simulink model "Gray_Binarization"  (R2013b)
settings: Solver=ode45  StartTime=0.0  StopTime=1000  RelTol=1e-3
InitFcn:
  | %% DSPBuilder Start
  | alt_dspbuilder_update_model(bdroot)
  | %% DSPBuilder End
libraries: allblocks_alteradspbuilder2 x44, simulink x3
settings Model: Creator=Given_Jiang  LastModifiedBy=Given_Jiang

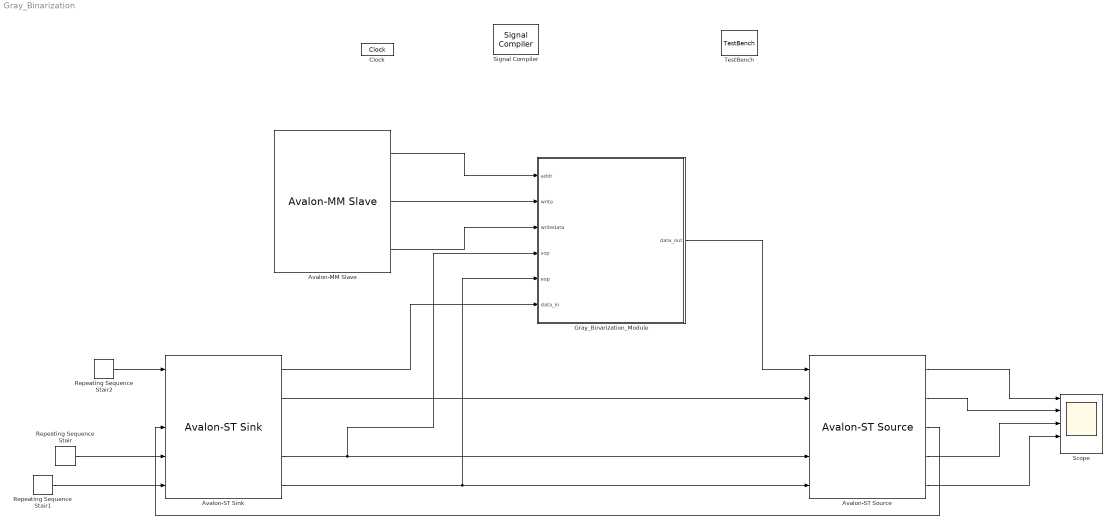
== system Gray_Binarization ==
  Avalon-MM Slave : allblocks_alteradspbuilder2/Avalon-MM Slave  iofile=E:\FPGA\SOC\Quartus\quartus\dsp_builder\design\VIP_LIB\Gray_Binarization\tb_Gray_Binarization\Gray%5FBinarization_Avalon-MM+Slave_address.salt,E:\FPGA\SOC\Quartus\quartus\dsp_builder\design\VIP_LIB\Gray_Binarization\tb_Gray_Binarization\Gray%5FBinarization_Avalon-MM+Slave_write.salt,E:\FPGA\SOC\Quartus\quartus\dsp_builder\design\VIP_LIB\Gray_Binarization\tb_Gray_Binarization\Gray%5FBinarization_Avalon-MM+Slave_writedata.salt,  SpecifyClock=off  addrWidth=2  addrAlignment=Dynamic  addrType=Write  BusType=Unsigned Integer  bwl=32  bwr=0  byteEnable=off  flowCtrl=off  pipeline=off  waitStateFormat=Fixed  readWaitStateCycles=0  writeWaitStateCycles=1  readLatencyFormat=Fixed  readLatencyCycles=0  burst=off  maxBurst=4  irq=off  receiveBeginTransfer=off  useChipSelect=off  externalType=Inferred  PORTTYPE=Output
  Avalon-ST Sink : allblocks_alteradspbuilder2/Avalon-ST Sink  iofile=E:\FPGA\SOC\Quartus\quartus\dsp_builder\design\VIP_LIB\Gray_Binarization\tb_Gray_Binarization\Gray%5FBinarization_Avalon-ST+Sink_data.salt,E:\FPGA\SOC\Quartus\quartus\dsp_builder\design\VIP_LIB\Gray_Binarization\tb_Gray_Binarization\Gray%5FBinarization_Avalon-ST+Sink_valid.salt,E:\FPGA\SOC\Quartus\quartus\dsp_builder\design\VIP_LIB\Gray_Binarization\tb_Gray_Binarization\Gray%5FBinarization_Avalon-ST+Sink_ready.capture,E:\FPGA\SOC\Quartus\quartus\dsp_builder\design\VIP_LIB\Gray_Binarization\tb_Gray_Binarization\Gray%5FBinarization_Avalon-ST+Sink_startofpacket.salt,E:\FPGA\SOC\Quartus\quartus\dsp_builder\design\VIP_LIB\Gray_Binarization\tb_Gray_Binarization\Gray%5FBinarization_Avalon-ST+Sink_endofpacket.salt,  SpecifyClock=off  BusType=Unsigned Integer  bwl=24  bwr=0  symbolWidth=8  symbolsPerBeat=3  numOfChannels=0  numOfErrorDescriptors=0  endOfPacket=on  startOfPacket=on  empty=off  readyLatency=1  externalType=Inferred  PORTTYPE=Output
  Avalon-ST Source : allblocks_alteradspbuilder2/Avalon-ST Source  iofile=E:\FPGA\SOC\Quartus\quartus\dsp_builder\design\VIP_LIB\Gray_Binarization\tb_Gray_Binarization\Gray%5FBinarization_Avalon-ST+Source_data.capture,E:\FPGA\SOC\Quartus\quartus\dsp_builder\design\VIP_LIB\Gray_Binarization\tb_Gray_Binarization\Gray%5FBinarization_Avalon-ST+Source_valid.capture,E:\FPGA\SOC\Quartus\quartus\dsp_builder\design\VIP_LIB\Gray_Binarization\tb_Gray_Binarization\Gray%5FBinarization_Avalon-ST+Source_ready.salt,E:\FPGA\SOC\Quartus\quartus\dsp_builder\design\VIP_LIB\Gray_Binarization\tb_Gray_Binarization\Gray%5FBinarization_Avalon-ST+Source_startofpacket.capture,E:\FPGA\SOC\Quartus\quartus\dsp_builder\design\VIP_LIB\Gray_Binarization\tb_Gray_Binarization\Gray%5FBinarization_Avalon-ST+Source_endofpacket.capture,  SpecifyClock=off  BusType=Unsigned Integer  bwl=24  bwr=0  symbolWidth=8  symbolsPerBeat=3  numOfChannels=0  numOfErrorDescriptors=0  endOfPacket=on  startOfPacket=on  empty=off  readyLatency=1  externalType=Inferred  PORTTYPE=Input
  Clock : allblocks_alteradspbuilder2/Clock  ClockPeriod=7.5  ClockPeriodUnit=ns  SampleTime=1  ResetLatency=0  ResetRegisterCascadeDepth=0  SimulationStartCycle=5  PhaseOffset=0  Reset=aclr  ResetType=Active Low  Export=off
  Gray_Binarization_Module : Subsystem
  Repeating Sequence Stair : simulink/Sources/Repeating Sequence Stair  OutValues=[1 0 0 0 1 0 0 0 0 0].'  tsamp=-1  OutMin=[]  OutMax=[]  OutDataTypeStr=double  OutputDataTypeScalingMode=double  OutDataType=fixdt(0,8)  ConRadixGroup=Best Precision: Vector-wise  OutScaling=2^-12
  Repeating Sequence Stair1 : simulink/Sources/Repeating Sequence Stair  OutValues=[0 0 0 1 0 0 0 0 0 1].'  tsamp=-1  OutMin=[]  OutMax=[]  OutDataTypeStr=double  OutputDataTypeScalingMode=double  OutDataType=fixdt(0,8)  ConRadixGroup=Best Precision: Vector-wise  OutScaling=2^-12
  Repeating Sequence Stair2 : simulink/Sources/Repeating Sequence Stair  OutValues=[15 101 102 103 0 65793 66305 255 255 1].'  tsamp=-1  OutMin=[]  OutMax=[]  OutDataTypeStr=double  OutputDataTypeScalingMode=double  OutDataType=fixdt(0,8)  ConRadixGroup=Best Precision: Vector-wise  OutScaling=2^-12
  Scope : Scope  NumInputPorts=5
      settings: YMin=-5~-5~-5~-5~-5  YMax=5~5~5~5~5
  Signal Compiler : allblocks_alteradspbuilder2/Signal Compiler  DeviceFamily=Cyclone V  DeviceName=AUTO  DisableEarlyHDLGeneration=off  EnableSignalTap=off  SignalTapDepth=128  UseBoardBlock=off  StpUseDefaultClock=on  StpClock=Clock  ExportDir=E:\FPGA\SOC\Quartus\quartus\dsp_builder
  TestBench : allblocks_alteradspbuilder2/TestBench  enable=on  advancedMode=on  modelSimGui=on  maxDisplayErrors=10  mismatchErrorLevel=Error  simdatafile=E:\FPGA\SOC\Quartus\quartus\dsp_builder\design\VIP_LIB\Gray_Binarization\tb_Gray_Binarization\Gray_Binarization.simdata.tcl
  wires:
  Avalon-ST Sink/2 -> Avalon-ST Source/2
  Avalon-ST Source/3 -> Avalon-ST Sink/3
  Avalon-ST Sink/4 -> Gray_Binarization_Module/4(sop), Avalon-ST Source/4
  Avalon-ST Sink/5 -> Gray_Binarization_Module/5(eop), Avalon-ST Source/5
  Avalon-ST Sink/1 -> Gray_Binarization_Module/6(data_in)
  Avalon-MM Slave/1 -> Gray_Binarization_Module/1(addr)
  Avalon-MM Slave/2 -> Gray_Binarization_Module/2(write)
  Avalon-MM Slave/3 -> Gray_Binarization_Module/3(writedata)
  Gray_Binarization_Module/1(data_out) -> Avalon-ST Source/1
  Repeating Sequence Stair/1 -> Avalon-ST Sink/4
  Repeating Sequence Stair1/1 -> Avalon-ST Sink/5
  Repeating Sequence Stair2/1 -> Avalon-ST Sink/1
  Avalon-ST Source/1 -> Scope/1
  Avalon-ST Source/2 -> Scope/2
  Avalon-ST Source/4 -> Scope/3
  Avalon-ST Source/5 -> Scope/4

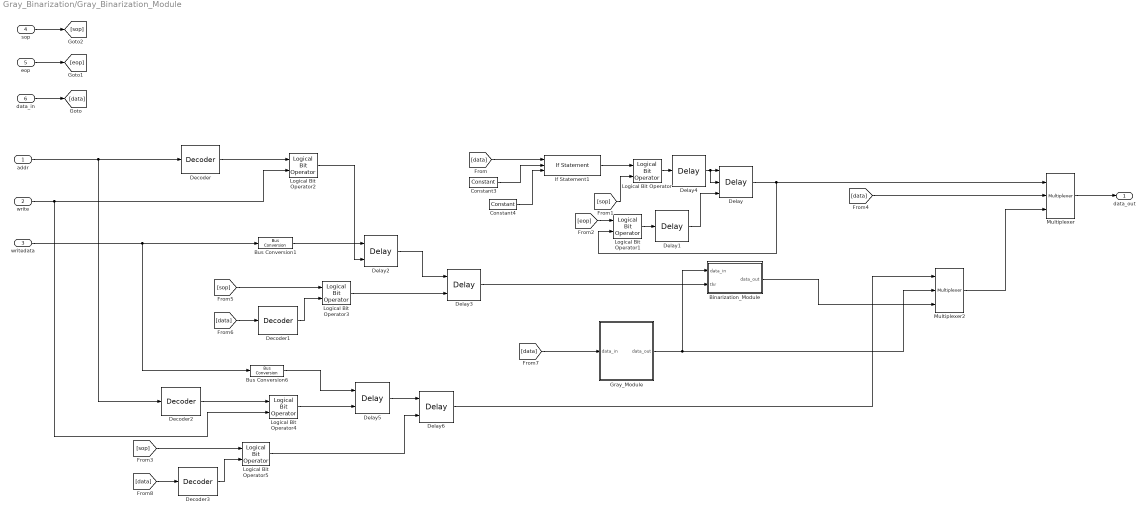
== system Gray_Binarization/Gray_Binarization_Module ==
  addr : Inport
  write : Inport  Port=2
  writedata : Inport  Port=3
  sop : Inport  Port=4
  eop : Inport  Port=5
  data_in : Inport  Port=6
  Binarization_Module : Subsystem
  Bus Conversion1 : allblocks_alteradspbuilder2/Bus Conversion  BusType=Unsigned Integer  ibwl=32  ibwr=1  bwl=8  bwr=1  bitToConnectToOutputLSB=0  round=off  saturate=off  pipeline_display=0
  Bus Conversion6 : allblocks_alteradspbuilder2/Bus Conversion  BusType=Unsigned Integer  ibwl=32  ibwr=1  bwl=1  bwr=1  bitToConnectToOutputLSB=0  round=off  saturate=off  pipeline_display=0
  Constant3 : allblocks_alteradspbuilder2/Constant  mask_cst=0  BusType=Unsigned Integer  bwl=24  bwr=0  roundMode=Truncate  satMode=Wrap  SpecifyClock=off  allowFloatingPointOverride=on  logOutputs=off  logFile=E:\FPGA\SOC\Quartus\quartus\dsp_builder\design\VIP_LIB\Gray_Binarization\tb_Gray_Binarization\Gray%5FBinarization_Gray%5FBinarization%5FModule_Constant3.fixedpointlog
  Constant4 : allblocks_alteradspbuilder2/Constant  mask_cst=15  BusType=Unsigned Integer  bwl=24  bwr=0  roundMode=Truncate  satMode=Wrap  SpecifyClock=off  allowFloatingPointOverride=on  logOutputs=off  logFile=E:\FPGA\SOC\Quartus\quartus\dsp_builder\design\VIP_LIB\Gray_Binarization\tb_Gray_Binarization\Gray%5FBinarization_Gray%5FBinarization%5FModule_Constant4.fixedpointlog
  Decoder : allblocks_alteradspbuilder2/Decoder  BusType=Unsigned Integer  bwl=2  bwr=2  registered=on  pipeline_display=1  value=2
  Decoder1 : allblocks_alteradspbuilder2/Decoder  BusType=Unsigned Integer  bwl=24  bwr=2  registered=off  pipeline_display=0  value=15
  Decoder2 : allblocks_alteradspbuilder2/Decoder  BusType=Unsigned Integer  bwl=2  bwr=2  registered=on  pipeline_display=1  value=1
  Decoder3 : allblocks_alteradspbuilder2/Decoder  BusType=Unsigned Integer  bwl=24  bwr=2  registered=off  pipeline_display=0  value=15
  Delay : allblocks_alteradspbuilder2/Delay  pipeline=1  pipeline_display=1  ClockPhase=1  use_ena=on  use_sclr=on  allowFloatingPointOverride=on  logOutputs=off  logFile=E:\FPGA\SOC\Quartus\quartus\dsp_builder\design\VIP_LIB\Gray_Binarization\tb_Gray_Binarization\Gray%5FBinarization_Gray%5FBinarization%5FModule_Delay.fixedpointlog  use_init=on  reset_value=0
  Delay1 : allblocks_alteradspbuilder2/Delay  pipeline=1  pipeline_display=1  ClockPhase=1  use_ena=off  use_sclr=off  allowFloatingPointOverride=on  logOutputs=off  logFile=E:\FPGA\SOC\Quartus\quartus\dsp_builder\design\VIP_LIB\Gray_Binarization\tb_Gray_Binarization\Gray%5FBinarization_Gray%5FBinarization%5FModule_Delay1.fixedpointlog  use_init=off  reset_value=0
  Delay2 : allblocks_alteradspbuilder2/Delay  pipeline=1  pipeline_display=1  ClockPhase=1  use_ena=on  use_sclr=off  allowFloatingPointOverride=on  logOutputs=off  logFile=E:\FPGA\SOC\Quartus\quartus\dsp_builder\design\VIP_LIB\Gray_Binarization\tb_Gray_Binarization\Gray%5FBinarization_Gray%5FBinarization%5FModule_Delay2.fixedpointlog  use_init=on  reset_value=127
  Delay3 : allblocks_alteradspbuilder2/Delay  pipeline=1  pipeline_display=1  ClockPhase=1  use_ena=on  use_sclr=off  allowFloatingPointOverride=on  logOutputs=off  logFile=E:\FPGA\SOC\Quartus\quartus\dsp_builder\design\VIP_LIB\Gray_Binarization\tb_Gray_Binarization\Gray%5FBinarization_Gray%5FBinarization%5FModule_Delay3.fixedpointlog  use_init=on  reset_value=127
  Delay4 : allblocks_alteradspbuilder2/Delay  pipeline=1  pipeline_display=1  ClockPhase=1  use_ena=off  use_sclr=off  allowFloatingPointOverride=on  logOutputs=off  logFile=E:\FPGA\SOC\Quartus\quartus\dsp_builder\design\VIP_LIB\Gray_Binarization\tb_Gray_Binarization\Gray%5FBinarization_Gray%5FBinarization%5FModule_Delay4.fixedpointlog  use_init=off  reset_value=0
  Delay5 : allblocks_alteradspbuilder2/Delay  pipeline=1  pipeline_display=1  ClockPhase=1  use_ena=on  use_sclr=off  allowFloatingPointOverride=on  logOutputs=off  logFile=E:\FPGA\SOC\Quartus\quartus\dsp_builder\design\VIP_LIB\Gray_Binarization\tb_Gray_Binarization\Gray%5FBinarization_Gray%5FBinarization%5FModule_Delay5.fixedpointlog  use_init=on  reset_value=0
  Delay6 : allblocks_alteradspbuilder2/Delay  pipeline=1  pipeline_display=1  ClockPhase=1  use_ena=on  use_sclr=off  allowFloatingPointOverride=on  logOutputs=off  logFile=E:\FPGA\SOC\Quartus\quartus\dsp_builder\design\VIP_LIB\Gray_Binarization\tb_Gray_Binarization\Gray%5FBinarization_Gray%5FBinarization%5FModule_Delay6.fixedpointlog  use_init=on  reset_value=0
  Gray_Module : Subsystem
  If Statement1 : allblocks_alteradspbuilder2/If Statement  user_inputs=3  if_expression=(a=b)&(a~c)  BusType=Unsigned Integer  bwl=24  bwr=0  pipeline_display=1  use_else_output=off  use_elseif_input=off
  Logical Bit Operator{,1..5} (6 alike) : allblocks_alteradspbuilder2/Logical Bit Operator  LogicalOperator=AND  user_inputs=2  pipeline_display=0
  Multiplexer : allblocks_alteradspbuilder2/Multiplexer  numInputs=2  pipeline=0  oneHot=off  pipeline_display=0  use_ena=off  use_aclr=off  allowFloatingPointOverride=on  logOutputs=off  logFile=E:\FPGA\SOC\Quartus\quartus\dsp_builder\design\VIP_LIB\Gray_Binarization\tb_Gray_Binarization\Gray%5FBinarization_Gray%5FBinarization%5FModule_Multiplexer.fixedpointlog
  Multiplexer2 : allblocks_alteradspbuilder2/Multiplexer  numInputs=2  pipeline=0  oneHot=off  pipeline_display=0  use_ena=off  use_aclr=off  allowFloatingPointOverride=on  logOutputs=off  logFile=E:\FPGA\SOC\Quartus\quartus\dsp_builder\design\VIP_LIB\Gray_Binarization\tb_Gray_Binarization\Gray%5FBinarization_Gray%5FBinarization%5FModule_Multiplexer2.fixedpointlog
  data_out : Outport
  wires:
  If Statement1/1 -> Logical Bit Operator/1
  Delay/1 -> Logical Bit Operator1/2, Multiplexer/1
  [data] -> If Statement1/1
  [sop] -> Logical Bit Operator/2
  Gray_Module/1(data_out) -> Multiplexer2/2, Binarization_Module/1(data_in)
  [data] -> Multiplexer/2
  Multiplexer/1 -> data_out/1
  Constant3/1 -> If Statement1/2
  Constant4/1 -> If Statement1/3
  [eop] -> Logical Bit Operator1/1
  Logical Bit Operator1/1 -> Delay1/1
  Delay1/1 -> Delay/3
  addr/1 -> Decoder2/1, Decoder/1
  Decoder/1 -> Logical Bit Operator2/1
  write/1 -> Logical Bit Operator4/2, Logical Bit Operator2/2
  [data] -> Decoder1/1
  [sop] -> Logical Bit Operator3/1
  Decoder1/1 -> Logical Bit Operator3/2
  Logical Bit Operator2/1 -> Delay2/2
  Delay2/1 -> Delay3/1
  Logical Bit Operator3/1 -> Delay3/2
  writedata/1 -> Bus Conversion6/1, Bus Conversion1/1
  Bus Conversion1/1 -> Delay2/1
  data_in/1 -> [data]
  eop/1 -> [eop]
  sop/1 -> [sop]
  Logical Bit Operator/1 -> Delay4/1
  Delay4/1 -> Delay/2, Delay/1
  [data] -> Gray_Module/1(data_in)
  Multiplexer2/1 -> Multiplexer/3
  Decoder2/1 -> Logical Bit Operator4/1
  Delay5/1 -> Delay6/1
  [data] -> Decoder3/1
  [sop] -> Logical Bit Operator5/1
  Decoder3/1 -> Logical Bit Operator5/2
  Logical Bit Operator5/1 -> Delay6/2
  Logical Bit Operator4/1 -> Delay5/2
  Bus Conversion6/1 -> Delay5/1
  Delay6/1 -> Multiplexer2/1
  Binarization_Module/1(data_out) -> Multiplexer2/3
  Delay3/1 -> Binarization_Module/2(thr)

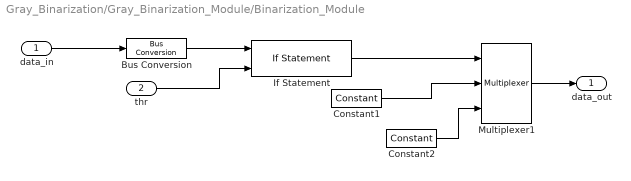
== system Gray_Binarization/Gray_Binarization_Module/Binarization_Module ==
  data_in : Inport
  thr : Inport  Port=2
  Bus Conversion : allblocks_alteradspbuilder2/Bus Conversion  BusType=Unsigned Integer  ibwl=24  ibwr=1  bwl=8  bwr=1  bitToConnectToOutputLSB=0  round=off  saturate=off  pipeline_display=0
  Constant1 : allblocks_alteradspbuilder2/Constant  mask_cst=0  BusType=Unsigned Integer  bwl=24  bwr=0  roundMode=Truncate  satMode=Wrap  SpecifyClock=off  allowFloatingPointOverride=on  logOutputs=off  logFile=E:\FPGA\SOC\Quartus\quartus\dsp_builder\design\VIP_LIB\Gray_Binarization\tb_Gray_Binarization\Gray%5FBinarization_Gray%5FBinarization%5FModule_Binarization%5FModule_Constant1.fixedpointlog
  Constant2 : allblocks_alteradspbuilder2/Constant  mask_cst=16777215  BusType=Unsigned Integer  bwl=24  bwr=0  roundMode=Truncate  satMode=Wrap  SpecifyClock=off  allowFloatingPointOverride=on  logOutputs=off  logFile=E:\FPGA\SOC\Quartus\quartus\dsp_builder\design\VIP_LIB\Gray_Binarization\tb_Gray_Binarization\Gray%5FBinarization_Gray%5FBinarization%5FModule_Binarization%5FModule_Constant2.fixedpointlog
  If Statement : allblocks_alteradspbuilder2/If Statement  user_inputs=2  if_expression=a>b  BusType=Unsigned Integer  bwl=8  bwr=0  pipeline_display=1  use_else_output=off  use_elseif_input=off
  Multiplexer1 : allblocks_alteradspbuilder2/Multiplexer  numInputs=2  pipeline=0  oneHot=off  pipeline_display=0  use_ena=off  use_aclr=off  allowFloatingPointOverride=on  logOutputs=off  logFile=E:\FPGA\SOC\Quartus\quartus\dsp_builder\design\VIP_LIB\Gray_Binarization\tb_Gray_Binarization\Gray%5FBinarization_Gray%5FBinarization%5FModule_Binarization%5FModule_Multiplexer1.fixedpointlog
  data_out : Outport
  wires:
  data_in/1 -> Bus Conversion/1
  thr/1 -> If Statement/2
  Bus Conversion/1 -> If Statement/1
  If Statement/1 -> Multiplexer1/1
  Constant1/1 -> Multiplexer1/2
  Constant2/1 -> Multiplexer1/3
  Multiplexer1/1 -> data_out/1

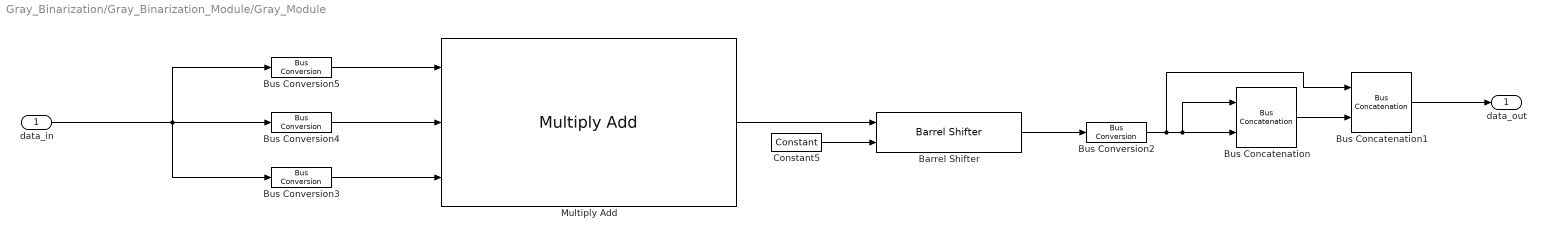
== system Gray_Binarization/Gray_Binarization_Module/Gray_Module ==
  data_in : Inport
  Barrel Shifter : allblocks_alteradspbuilder2/Barrel Shifter  BusType=Unsigned Integer  bwl=18  bwr=8  pipeline=off  infer_distance=off  distance_length=4  ShiftDirection=Shift right  use_ena=off  use_aclr=off  UseDedicatedCircuitry=off  pipeline_display=0  allowFloatingPointOverride=on  logOutputs=off  logFile=E:\FPGA\SOC\Quartus\quartus\dsp_builder\design\VIP_LIB\Gray_Binarization\tb_Gray_Binarization\Gray%5FBinarization_Gray%5FBinarization%5FModule_Gray%5FModule_Barrel+Shifter.fixedpointlog
  Bus Concatenation : allblocks_alteradspbuilder2/Bus Concatenation  isSigned=off  awidth=8  bwidth=8  pipeline_display=0
  Bus Concatenation1 : allblocks_alteradspbuilder2/Bus Concatenation  isSigned=off  awidth=8  bwidth=16  pipeline_display=0
  Bus Conversion2 : allblocks_alteradspbuilder2/Bus Conversion  BusType=Unsigned Integer  ibwl=18  ibwr=1  bwl=8  bwr=1  bitToConnectToOutputLSB=0  round=off  saturate=off  pipeline_display=0
  Bus Conversion3 : allblocks_alteradspbuilder2/Bus Conversion  BusType=Unsigned Integer  ibwl=24  ibwr=1  bwl=8  bwr=1  bitToConnectToOutputLSB=0  round=off  saturate=off  pipeline_display=0
  Bus Conversion4 : allblocks_alteradspbuilder2/Bus Conversion  BusType=Unsigned Integer  ibwl=24  ibwr=1  bwl=8  bwr=1  bitToConnectToOutputLSB=8  round=off  saturate=off  pipeline_display=0
  Bus Conversion5 : allblocks_alteradspbuilder2/Bus Conversion  BusType=Unsigned Integer  ibwl=24  ibwr=1  bwl=8  bwr=1  bitToConnectToOutputLSB=16  round=off  saturate=off  pipeline_display=0
  Constant5 : allblocks_alteradspbuilder2/Constant  mask_cst=8  BusType=Unsigned Integer  bwl=4  bwr=0  roundMode=Truncate  satMode=Wrap  SpecifyClock=off  allowFloatingPointOverride=on  logOutputs=off  logFile=E:\FPGA\SOC\Quartus\quartus\dsp_builder\design\VIP_LIB\Gray_Binarization\tb_Gray_Binarization\Gray%5FBinarization_Gray%5FBinarization%5FModule_Gray%5FModule_Constant5.fixedpointlog
  Multiply Add : allblocks_alteradspbuilder2/Multiply Add  multipliers=3  BusType=Unsigned Integer  bwl=8  bwr=0  direction=Add Add  pipeline_register=No Register  pipeline_display=0  use_constants=on  constants=[76 150 30]  UseDedicatedCircuitry=on  use_ena=off  use_aclr=off  allowFloatingPointOverride=on  logOutputs=off  logFile=E:\FPGA\SOC\Quartus\quartus\dsp_builder\design\VIP_LIB\Gray_Binarization\tb_Gray_Binarization\Gray%5FBinarization_Gray%5FBinarization%5FModule_Gray%5FModule_Multiply+Add.fixedpointlog
  data_out : Outport
  wires:
  data_in/1 -> Bus Conversion3/1, Bus Conversion4/1, Bus Conversion5/1
  Barrel Shifter/1 -> Bus Conversion2/1
  Bus Conversion2/1 -> Bus Concatenation1/1, Bus Concatenation/1, Bus Concatenation/2
  Bus Concatenation/1 -> Bus Concatenation1/2
  Constant5/1 -> Barrel Shifter/2
  Bus Conversion5/1 -> Multiply Add/1
  Bus Conversion4/1 -> Multiply Add/2
  Bus Conversion3/1 -> Multiply Add/3
  Multiply Add/1 -> Barrel Shifter/1
  Bus Concatenation1/1 -> data_out/1
